simulink model "bench_tms"  (R2024b)
settings: Solver=daessc  StartTime=0.0  StopTime=7200  MaxStep=1  RelTol=1e-3
libraries: loco_native_lib x2
settings Model: Creator=BillBeverley  LastModifiedBy=BillBeverley

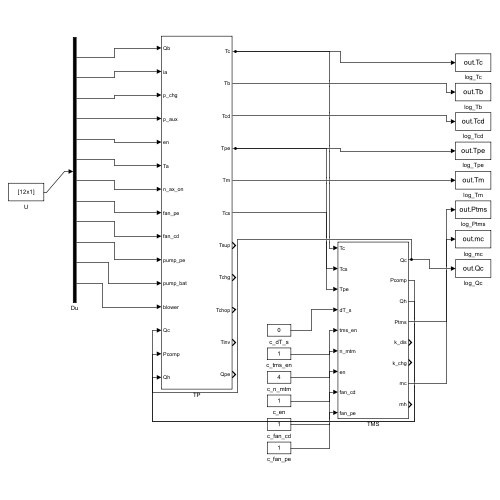
[thumbnail: Simulink's stored preview of the top-level diagram]
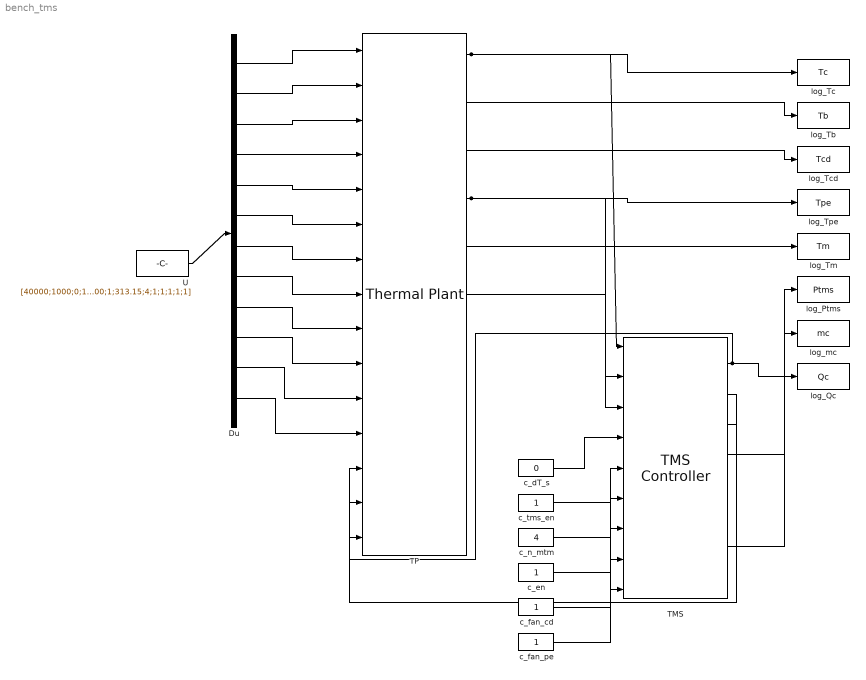
== system bench_tms ==
  Du : Demux  Outputs=12
  TMS : loco_native_lib/TMS Controller  TH=P.th  Ts=0.1
  TP : loco_native_lib/Thermal Plant  TH=P.th  f_ram=0.2
  U : Constant  Value=[40000;1000;0;100000;1;313.15;4;1;1;1;1;1]
  c_dT_s : Constant  Value=0
  c_en : Constant
  c_fan_cd : Constant
  c_fan_pe : Constant
  c_n_mtm : Constant  Value=4
  c_tms_en : Constant
  log_Ptms : ToWorkspace  VariableName=Ptms  SaveFormat=Timeseries  SampleTime=-1
  log_Qc : ToWorkspace  VariableName=Qc  SaveFormat=Timeseries  SampleTime=-1
  log_Tb : ToWorkspace  VariableName=Tb  SaveFormat=Timeseries  SampleTime=-1
  log_Tc : ToWorkspace  VariableName=Tc  SaveFormat=Timeseries  SampleTime=-1
  log_Tcd : ToWorkspace  VariableName=Tcd  SaveFormat=Timeseries  SampleTime=-1
  log_Tm : ToWorkspace  VariableName=Tm  SaveFormat=Timeseries  SampleTime=-1
  log_Tpe : ToWorkspace  VariableName=Tpe  SaveFormat=Timeseries  SampleTime=-1
  log_mc : ToWorkspace  VariableName=mc  SaveFormat=Timeseries  SampleTime=-1
  wires:
  U/1 -> Du/1
  Du/1 -> TP/1
  Du/2 -> TP/2
  Du/3 -> TP/3
  Du/4 -> TP/4
  Du/5 -> TP/5
  Du/6 -> TP/6
  Du/7 -> TP/7
  Du/8 -> TP/8
  Du/9 -> TP/9
  Du/10 -> TP/10
  Du/11 -> TP/11
  Du/12 -> TP/12
  TMS/1 -> TP/13, log_Qc/1
  TMS/2 -> TP/14
  TMS/3 -> TP/15
  TP/1 -> TMS/1, log_Tc/1
  TP/6 -> TMS/2
  TP/4 -> TMS/3, log_Tpe/1
  c_dT_s/1 -> TMS/4
  c_tms_en/1 -> TMS/5
  c_n_mtm/1 -> TMS/6
  c_en/1 -> TMS/7
  c_fan_cd/1 -> TMS/8
  c_fan_pe/1 -> TMS/9
  TP/2 -> log_Tb/1
  TP/3 -> log_Tcd/1
  TP/5 -> log_Tm/1
  TMS/4 -> log_Ptms/1
  TMS/7 -> log_mc/1
